simulink model "environment"  (R2024a)
settings: configuration reference "standardSILConfiguraitonParams" (kept outside this file)
settings Model: Creator=jerem  LastModifiedBy=jerem
settings ConfigSetRef: SourceName=standardSILConfiguraitonParams  SourceLocation=Base Workspace

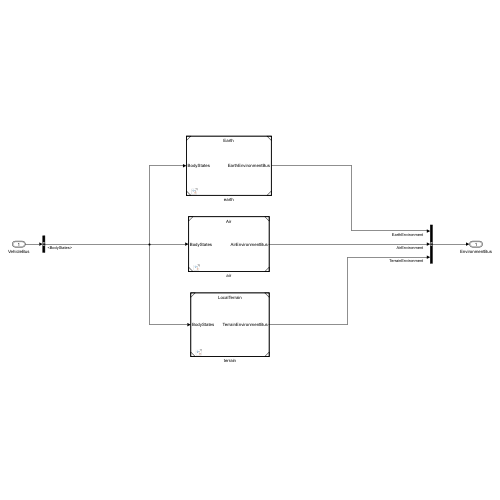
[thumbnail: Simulink's stored preview of the top-level diagram]
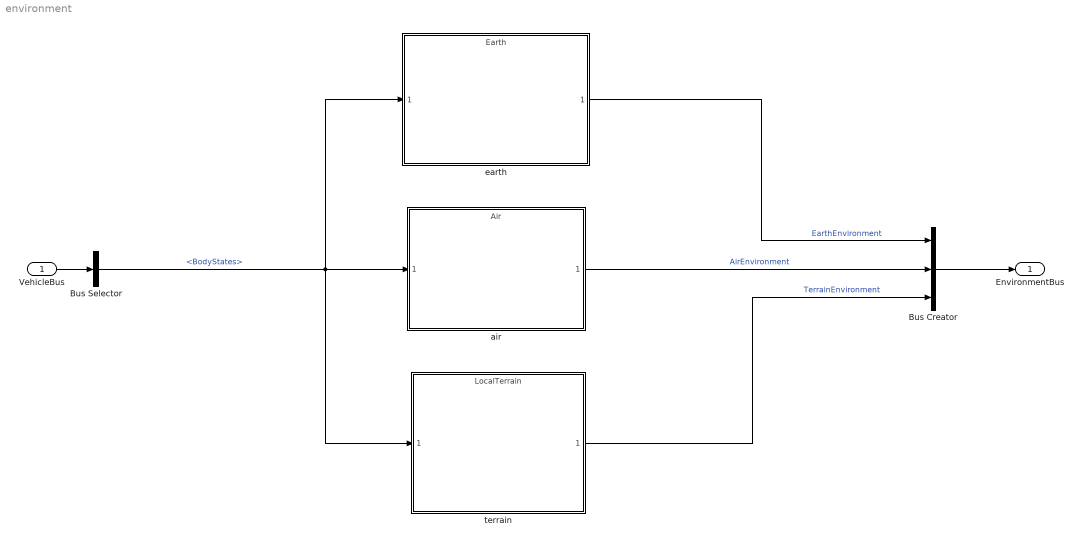
== system environment ==
  VehicleBus : Inport  OutDataTypeStr=Bus: VehicleBus
  Bus Creator : BusCreator  Inputs=3
  Bus Selector : BusSelector  OutputSignals=BodyStates
  air : ModelReference  ModelNameDialog=Air.slx  SimulationMode=Normal  ModelReferenceVersion=1.42
  earth : ModelReference  ModelNameDialog=Earth.slx  SimulationMode=Normal  ModelReferenceVersion=1.20
  terrain : ModelReference  ModelNameDialog=LocalTerrain.slx  SimulationMode=Normal  ModelReferenceVersion=1.6
  EnvironmentBus : Outport  OutDataTypeStr=Bus: EnvironmentBus
  wires:
  earth/1 -> Bus Creator/1  "EarthEnvironment"
  Bus Creator/1 -> EnvironmentBus/1
  terrain/1 -> Bus Creator/3  "TerrainEnvironment"
  VehicleBus/1 -> Bus Selector/1
  Bus Selector/1 -> air/1, terrain/1, earth/1  "<BodyStates>"
  air/1 -> Bus Creator/2  "AirEnvironment"
